simulink model "Blok_Diagram_RealTime"  (R2026a)
settings: Solver=FixedStepDiscrete  StopTime=300  FixedStep=512/44100
values from neighbouring files (symbols this model uses):
  cfgData = struct()    [precompute_cfg.m]
libraries: dspvision x2, dspsnks4 x1
settings Model: SimulationMode=accelerator  Creator=ASUS  LastModifiedBy=ASUS

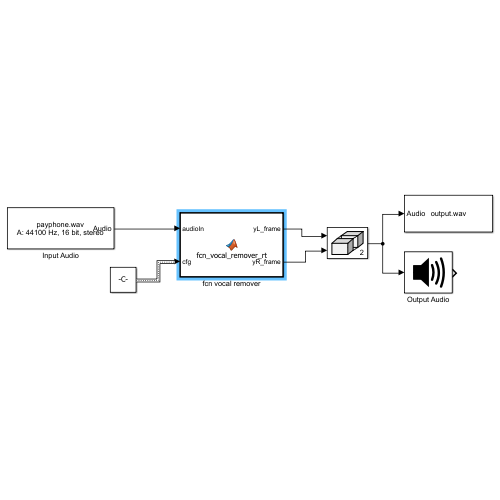
[thumbnail: Simulink's stored preview of the top-level diagram]
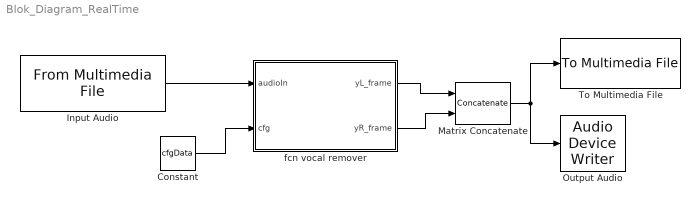
== system Blok_Diagram_RealTime ==
  Constant : Constant  Value=cfgData  OutDataTypeStr=Bus: slBus1
  Input Audio : dspvision/From Multimedia File  inputFilename=D:\Nathanael\Telkom University\Semester 6\Kerja Praktek\ICDEC\Vocal Remover Phase MATLAB\payphone.wav  readRange=[1 Inf]  loop=on  numPlays=inf  outputStreams=Audio only  videoDataType=single  audioDataType=double  inheritSampleTime=on  userDefinedSampleTime=1/30  noAudioOutput=off  isIntensityVideo=off  fourcc=RGB  colorVideoFormat=Separate color signals  outputEOF=off  dataOrg=Column-major  audioFrameSize=512  computeAudioFrameSize=off  outSamplingMode=Sample based
      settings: LibrarySourceBlock=audiosources/From Multimedia File
  Matrix Concatenate : Concatenate  Mode=Multidimensional array  ConcatenateDimension=2
  Output Audio : dspsnks4/Audio Device Writer  Driver=DirectSound  Device=Default  InheritSampleRate=off  SampleRate=44100  BitDepth=16-bit integer  BufferSize=4096  NumBuffers=10  DefaultOutputChannelMapping=on  OutputChannelMapping=1:2  OutputNumUnderrunSamples=on  DriverIdx=1  DeviceWarnFlag=''
  To Multimedia File : dspvision/To Multimedia File  outputFilename=output.wav  streamSelection=Audio only  videoCompressor=None (uncompressed)  audioCompressor=None (uncompressed)  imagePorts=Separate color signals  fileType=WAV  audioDatatype=16-bit integer  fourcc=RGB  audioBitRate=128  audioQuality=75  videoQuality=75  mj2000CompFactor=10
      settings: LibrarySourceBlock=audiosinks/To Multimedia File
  fcn vocal remover : MATLAB Function  TreatAsAtomicUnit=on
  wires:
  Input Audio/1 -> fcn vocal remover/1(audioIn)
  Constant/1 -> fcn vocal remover/2(cfg)
  fcn vocal remover/1(yL_frame) -> Matrix Concatenate/1
  fcn vocal remover/2(yR_frame) -> Matrix Concatenate/2
  Matrix Concatenate/1 -> To Multimedia File/1, Output Audio/1

== matlab function Blok_Diagram_RealTime/fcn vocal remover ==
  data: audioIn input; yL_frame output; cfg input Bus: slBus1; yR_frame output
function [yL_frame, yR_frame] = fcn_vocal_remover_rt(audioIn, cfg) %#codegen
% FCN_VOCAL_REMOVER_RT
% Isi 1 MATLAB Function block Simulink, menggantikan 4 block lama
% (fcn_preprocessing, fcn_core, fcn_postprocessing, fcn_apply_istft).
%
% Input:
%   audioIn : matriks [hop x 2] (kolom 1 = L, kolom 2 = R), langsung dari
%             source audio (misal "From Multimedia File", frame=512,
%             stereo) -- TIDAK PERLU Demux/Selector, pemecahan L/R
%             dilakukan di dalam block ini.
%   cfg     : struct hasil precompute_cfg.m (semua numerik, sudah
%             masuk ke block via Constant/Bus -- BUKAN dihitung di
%             sini, supaya discretize()/unique() tidak pernah kena
%             code generation).
% Output:
%   yL_frame, yR_frame : hop-length sample output siap diputar.
%
% CATATAN CODEGEN:
% - Semua state persistent harus di-set ukuran TETAP sejak awal (tidak ada
%   growing array, tidak ada isfield check).
% - Tidak ada cell array (cfg.bandMask sudah matriks N x numBands).
% - corr/xcorr/discretize/unique/conv2/prctile/medfilt1 SUDAH TIDAK ADA
%   di file ini.

% [FIX CODEGEN] N, hop, numBands HARUS konstanta compile-time (literal),
% TIDAK BOLEH dibaca dari cfg (bus/data runtime) -- karena dipakai untuk
% menentukan ukuran array (zeros(N,1) dst). Kalau diambil dari cfg.N,
% Coder anggap ukurannya bisa berubah -> semua array jadi variable-size
% -> output block juga ikut variable-size.
%
% Nilai berikut sudah dikonfirmasi cocok dgn cfgData kamu:
%   cfgData.N=2048, cfgData.hop=512, cfgData.numBands=34,
%   cfgData.lagMin=44, cfgData.lagMax=551
N   = 2048;
hop = 512;
numBands = 34;

L_hop = audioIn(:,1);
R_hop = audioIn(:,2);

%% --- PERSISTENT STATE (setara discrete state Simulink) ---
persistent inBufL inBufR outBufL outBufR winSumBuf
persistent ziL ziR
persistent corrLR_ELR corrLR_EL2 corrLR_ER2
persistent fluxMean fluxVar magSumPrev
persistent bandPhasorBuf bandPhasorBufCount
persistent vlBuf vlBufCount
persistent gainBandPrev gainMedianBuf
persistent fracHighPLV_run
persistent holdCounter
persistent isInit

if isempty(isInit)
    inBufL = zeros(N,1);  inBufR = zeros(N,1);
    outBufL = zeros(N,1); outBufR = zeros(N,1);
    winSumBuf = zeros(N,1);
    ziL = 0; ziR = 0;
    corrLR_ELR = 0; corrLR_EL2 = eps; corrLR_ER2 = eps;
    fluxMean = 0; fluxVar = 0; magSumPrev = 0;
    bandPhasorBuf = complex(zeros(numBands, cfg.p_timeSmoothFrames));
    bandPhasorBufCount = 0;
    vlBuf = zeros(1, cfg.p_vlSmoothFrames);
    vlBufCount = 0;
    gainBandPrev = ones(numBands,1);
    gainMedianBuf = ones(numBands, cfg.p_postMedianFrames);
    fracHighPLV_run = zeros(numBands,1);
    holdCounter = 0;
    isInit = true;
end

L_hop = L_hop(:); R_hop = R_hop(:);

%% --- BUFFER INPUT (sliding window causal) ---
inBufL = [inBufL(hop+1:end); L_hop];
inBufR = [inBufR(hop+1:end); R_hop];

%% --- DC REMOVAL (vectorized filter dgn state carry) ---
a = cfg.R_dc;
[Lc, ziL] = filter([1 -1], [1 -a], L_hop, ziL);
[Rc, ziR] = filter([1 -1], [1 -a], R_hop, ziR);

%% --- KORELASI L-R RUNNING (EMA, ganti corr() global) ---
alpha = cfg.corrLR_alpha;
corrLR_ELR = (1-alpha)*corrLR_ELR + alpha*mean(Lc.*Rc);
corrLR_EL2 = (1-alpha)*corrLR_EL2 + alpha*mean(Lc.^2);
corrLR_ER2 = (1-alpha)*corrLR_ER2 + alpha*mean(Rc.^2);
corrLR = corrLR_ELR / max(eps, sqrt(corrLR_EL2 * corrLR_ER2));
corrLR = max(-1, min(1, corrLR));

depthScale = 1.0;
if corrLR > cfg.p_corrLRWarnThresh
    frac = (corrLR - cfg.p_corrLRWarnThresh) / max(eps, (cfg.p_corrLRHardThresh - cfg.p_corrLRWarnThresh));
    frac = min(1, max(0, frac));
    depthScale = 1.0 - frac * (1.0 - cfg.p_minDepthScale);
end
depthNow = cfg.p_depth * depthScale;
if corrLR > cfg.p_corrLRWarnThresh
    fracFloor = (corrLR - cfg.p_corrLRWarnThresh) / max(eps, (cfg.p_corrLRHardThresh - cfg.p_corrLRWarnThresh));
    fracFloor = min(1, max(0, fracFloor));
    gainFloor = cfg.p_gainFloorBase + fracFloor * (cfg.p_gainFloorMono - cfg.p_gainFloorBase);
else
    gainFloor = cfg.p_gainFloorBase;
end

%% --- STFT FRAME TUNGGAL ---
frameL = inBufL .* cfg.win;
frameR = inBufR .* cfg.win;
XL = fft(frameL, N);
XR = fft(frameR, N);

%% --- PITCH (autocorrelation manual, sudah codegen-safe) ---
mono = (inBufL + inBufR)/2;
frame = mono .* cfg.win;
frame = frame - mean(frame);
% [FIX CODEGEN] sama seperti N/hop/numBands -- lagMin/lagMax dipakai utk
% ukuran array (numLags), jadi HARUS konstanta literal, bukan dari cfg.
% Nilai default ini utk fs=44100, pitchFmin=80, pitchFmax=1000:
%   lagMin = round(44100/1000) = 44
%   lagMax = round(44100/80)   = 551
% GANTI kalau parameter pitch/fs kamu beda (cek cfgData.lagMin/lagMax).
lagMin = 44; lagMax = 551;

frameLen = length(frame);
energy0 = sum(frame.^2) + eps;
numLags = lagMax - lagMin + 1;
segment = zeros(numLags, 1);
for li = 1:numLags
    lag = lagMin + li - 1;
    if lag < frameLen
        aSeg = frame(1:frameLen-lag);
        bSeg = frame(1+lag:frameLen);
        segment(li) = sum(aSeg .* bSeg) / energy0;
    end
end

if all(segment==0)
    clarity = 0; bestLag = 0;
else
    [clarity, relLag] = max(segment);
    bestLag = lagMin + relLag - 1;
end
vlRaw = max(0, clarity);
if bestLag > 0
    f0 = cfg.fs / bestLag;
else
    f0 = 0;
end
if vlRaw < cfg.p_clarityFloor
    vlRaw = 0;
end

if vlRaw > cfg.p_clarityFloor
    holdCounter = cfg.p_holdFrames;
elseif holdCounter > 0
    holdCounter = holdCounter - 1;
    vlRaw = max(vlRaw, cfg.p_holdLikelihoodValue);
end

vlBuf = [vlBuf(2:end), vlRaw];
vlBufCount = min(cfg.p_vlSmoothFrames, vlBufCount + 1);
vocalLikelihood = sum(vlBuf(end-vlBufCount+1:end)) / vlBufCount;
vocalLikelihood = min(1, vocalLikelihood);
vocalLikelihood = max(cfg.p_vocalLikelihoodFloor, vocalLikelihood);

%% --- PLV PER BAND (vektorisasi matriks, ganti loop cell bandBins) ---
% [FIX SIMULINK] cfg.bandMask: N x numBands (0/1). Perkalian matriks ini
% JUGA lebih ramah untuk implementasi HW/DSP chip dibanding loop+find().
unitPhasor = exp(1j*(angle(XL) - angle(XR)));
magWeight  = (abs(XL) + abs(XR))/2;

wp = unitPhasor .* magWeight;                 % N x 1 (complex)
numPhasor = cfg.bandMask' * wp;               % numBands x 1 (complex)
denPhasor = cfg.bandMask' * magWeight + eps;  % numBands x 1
bandMeanPhasorRaw = numPhasor ./ denPhasor;
bandMeanPhasorRaw(cfg.isProtectedBand > 0.5) = 0;

bandPhasorBuf = [bandPhasorBuf(:,2:end), bandMeanPhasorRaw];
bandPhasorBufCount = min(cfg.p_timeSmoothFrames, bandPhasorBufCount + 1);
bandMeanPhasorSmooth = sum(bandPhasorBuf(:, end-bandPhasorBufCount+1:end), 2) / bandPhasorBufCount;

PLVband = abs(bandMeanPhasorSmooth);
IPDband = angle(bandMeanPhasorSmooth);

%% --- RISK PER-BAND (EMA, ganti mean() global) ---
isHighPLVnow = double(PLVband > cfg.p_perBandRiskThresh);
ralpha = cfg.risk_alpha;
fracHighPLV_run = (1-ralpha)*fracHighPLV_run + ralpha*isHighPLVnow;

riskExcess = max(0, fracHighPLV_run - cfg.p_perBandRiskMinFrac) ./ max(eps, 1 - cfg.p_perBandRiskMinFrac);
riskExcess = min(1, riskExcess);
isCandidateBand = (cfg.boostMask < 0.5) & (cfg.isProtectedBand < 0.5);
riskProtectFactor = ones(numBands,1);
riskProtectFactor(isCandidateBand) = 1 - riskExcess(isCandidateBand) * (1 - cfg.p_perBandRiskProtectMin);

depthProfile = depthNow * (1 + cfg.boostRamp * (cfg.p_vocalBoostFactor - 1));
depthProfile = min(1, depthProfile);
depthProfile = depthProfile .* riskProtectFactor;

PLVbandWarped = PLVband .^ cfg.p_plvGamma;
centerScoreBand = PLVbandWarped .* exp(-(IPDband.^2) ./ (2*cfg.sigmaIPDperBand.^2));
centerScoreBand(PLVband < cfg.p_plvFloor) = 0;

%% --- HARMONIC SUPPORT (1 frame) ---
harmonicSupport = 0;
if f0 > 0
    supportVals = nan(1, cfg.p_maxHarmonics);
    cnt = 0;
    fmax = cfg.fs/2;
    for k = 1:cfg.p_maxHarmonics
        fk = f0*k;
        if fk > fmax, break; end
        bIdxArr = find(cfg.bandEdges(1:end-1) <= fk & cfg.bandEdges(2:end) > fk, 1);
        if isempty(bIdxArr)
            continue;
        end
        bIdx = bIdxArr(1);   % [FIX CODEGEN] paksa scalar, hindari logical op non-scalar
        if cfg.isProtectedBand(bIdx) > 0.5
            continue;
        end
        bandWidth = cfg.bandEdges(bIdx+1) - cfg.bandEdges(bIdx);
        distFromEdge = min(fk - cfg.bandEdges(bIdx), cfg.bandEdges(bIdx+1) - fk);
        if distFromEdge >= cfg.p_harmonicTolFrac * bandWidth * 0.5
            cnt = cnt + 1;
            supportVals(cnt) = centerScoreBand(bIdx);
        end
    end
    if cnt > 0
        harmonicSupport = mean(supportVals(1:cnt));
    end
end
vocalLikelihood = min(1, vocalLikelihood + cfg.p_harmonicBoostMax * harmonicSupport);

%% --- GATE + GAIN MENTAH ---
vlBlend = (1 - cfg.p_gatingStrength) + cfg.p_gatingStrength * vocalLikelihood;
centerScoreBand = centerScoreBand * vlBlend;
gainBandRaw = 1 - depthProfile .* centerScoreBand;

%% --- TRANSIENT PROTECTION (adaptive threshold, ganti prctile) ---
magSumNow = sum(abs(XL) + abs(XR));
flux = max(0, magSumNow - magSumPrev);
magSumPrev = magSumNow;

falpha = cfg.flux_alpha;
prevMean = fluxMean;
fluxMean = (1-falpha)*prevMean + falpha*flux;
fluxVar  = (1-falpha)*fluxVar + falpha*(flux-prevMean)^2;
fluxStd = sqrt(max(0,fluxVar));
fluxThresh = fluxMean + cfg.p_transientKStd * fluxStd;
isTransient = flux > fluxThresh;

gainBandRaw = gainBandRaw + (1-gainBandRaw) * (cfg.p_transientProtectAmount * isTransient);

%% --- ATTACK/RELEASE ---
gainBandNow = zeros(numBands,1);
for b = 1:numBands
    if gainBandRaw(b) < gainBandPrev(b)
        coef = cfg.attackCoef;
    else
        coef = cfg.releaseCoef;
    end
    gainBandNow(b) = coef*gainBandPrev(b) + (1-coef)*gainBandRaw(b);
end
gainBandNow = max(gainFloor, gainBandNow);
gainBandPrev = gainBandNow;

% Causal median filter (ganti medfilt1)
gainMedianBuf = [gainMedianBuf(:,2:end), gainBandNow];
gainBandPost = median(gainMedianBuf, 2);

%% --- PETAKAN GAIN & TERAPKAN (vektorisasi, ganti loop cell bandBins) ---
effectiveGainPerBand = cfg.protectGain .* gainBandPost + (1 - cfg.protectGain) * 1;
effectiveGainPerBand(cfg.isProtectedBand > 0.5) = 1;   % band terproteksi -> gain 1
gainMap = cfg.bandMask * effectiveGainPerBand;          % N x 1

YL = XL .* gainMap;
YR = XR .* gainMap;

frameOutL = real(ifft(YL)) .* cfg.win;
frameOutR = real(ifft(YR)) .* cfg.win;

%% --- OVERLAP-ADD OUTPUT ---
outBufL = outBufL + frameOutL;
outBufR = outBufR + frameOutR;
winSumBuf = winSumBuf + cfg.win.^2;

wsOut = winSumBuf(1:hop);
wsOut(wsOut < 1e-8) = 1;
yL_frame = outBufL(1:hop) ./ wsOut;
yR_frame = outBufR(1:hop) ./ wsOut;

outBufL = [outBufL(hop+1:end); zeros(hop,1)];
outBufR = [outBufR(hop+1:end); zeros(hop,1)];
winSumBuf = [winSumBuf(hop+1:end); zeros(hop,1)];

end
